simulink model "ADCS_Software"  (R2025b)
settings: Solver=FixedStepDiscrete  StartTime=0.0  StopTime=10.0  RelTol=1e-3
undefined symbols (not defined in the file or in its folder): D1, P
settings Model: OrderFunctionsByDependency=on  Creator=eyrns  LastModifiedBy=eyrns
settings OptimizationCC: DefaultParameterBehavior=Inlined  EnhancedBackFolding=on  PassReuseOutputArgsAs=Individual arguments  ZeroExternalMemoryAtStartup=off  ZeroInternalMemoryAtStartup=off  OptimizeBlockOrder=speed  DifferentSizesBufferReuse=on  OptimizationCustomize=off  EfficientTunableParamExpr=on
settings DebuggingCC: ParameterTunabilityLossMsg=error
settings SFSimCC: MATLABDynamicMemAlloc=off
settings RTWCC: SystemTargetFile=ert.tlc  TemplateMakefile=ert_default_tmf  Description=Embedded Coder
settings CodeAppCC: ForceParamTrailComments=on  IgnoreCustomStorageClasses=off  OperatorAnnotations=on  SimulinkDataObjDesc=on  SFDataObjDesc=on  InsertBlockDesc=on
settings ERTTargetCC: ERTCustomFileTemplate=example_file_process.tlc  TargetLangStandard=C99 (ISO)  GenerateSampleERTMain=on

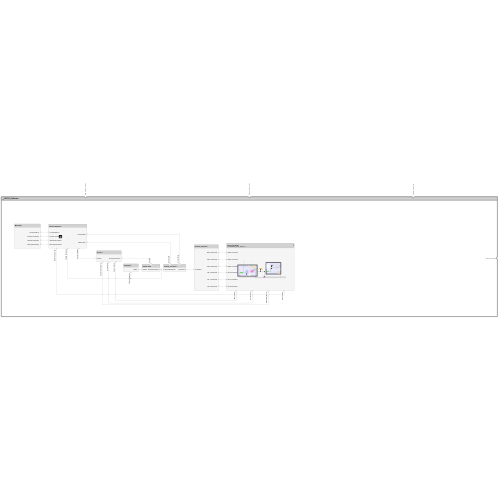
[thumbnail: Simulink's stored preview of the top-level diagram]
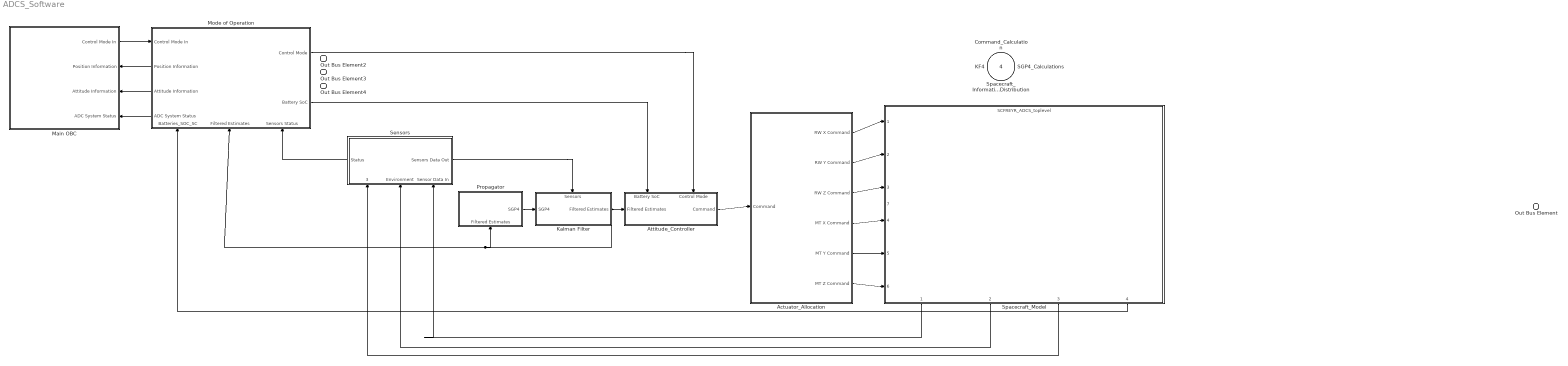
== system ADCS_Software ==
  Spacecraft_Information_Distribution : Inport  OutputFunctionCall=on
  Command_Calculation : Inport  Port=2  OutputFunctionCall=on
  SGP4_Calculations : Inport  Port=3  OutputFunctionCall=on
  KF4 : Inport  Port=4  OutputFunctionCall=on
  Actuator_Allocation : Subsystem
      settings: PortSchema="{\"entries\":[{\"content\":{\"headerSize\":26,\"margin\":15,\"minimumSpacing\":25,\"sides\":[{\"content\":{\"connectorIds\":[\"In1\"]},\"type\":\"ConnectorPlacement.EquallySpacedRectSide\",\"uuid\":\"256b1764-5093-40b4-a299-a96bc66f9c34\"},{\"content\":{\"connectorIds\":[\"Out1\",\"Out2\",\"Out3\",\"Out4\",\"Out5\",\"Out6\"],\"side\":\"RIGHT\"},\"type\":\"ConnectorPlacement.EquallySpacedRectSide\",\"uuid\":\"2deaa205-b527-45f3-83a3-1336b8d1b07d\"},{\"content\":{\"side\":\"TOP\"},\"type\":\"ConnectorPlacement.EquallySpacedRectSide\",\"uuid\":\"e475b6ad-a743-494b-935c-e32dd19b98b9\"}]},\"type\":\"ConnectorPlacement.EquallySpacedConnector\",\"uuid\":\"8ae79be5-f0b0-4f7e-ba91-8d68681c267d\"}],\"packageUris\":[\"http://schema.mathworks.com/mf0/Connector/R2020b\"],\"version\":\"1.0\"}"
  Attitude_Controller : Subsystem
      settings: PortSchema="{\"entries\":[{\"content\":{\"headerSize\":26,\"margin\":15,\"minimumSpacing\":25,\"sides\":[{\"content\":{\"connectorIds\":[\"In2\"]},\"type\":\"ConnectorPlacement.EquallySpacedRectSide\",\"uuid\":\"256b1764-5093-40b4-a299-a96bc66f9c34\"},{\"content\":{\"connectorIds\":[\"Out1\"],\"side\":\"RIGHT\"},\"type\":\"ConnectorPlacement.EquallySpacedRectSide\",\"uuid\":\"2deaa205-b527-45f3-83a3-1336b8d1b07d\"},{\"content\":{\"connectorIds\":[\"In1\",\"In3\"],\"side\":\"TOP\"},\"type\":\"ConnectorPlacement.EquallySpacedRectSide\",\"uuid\":\"e475b6ad-a743-494b-935c-e32dd19b98b9\"},{\"content\":{\"side\":\"BOTTOM\"},\"type\":\"ConnectorPlacement.EquallySpacedRectSide\",\"uuid\":\"40b931e7-0f08-4302-b6a2-74d313a26b2a\"}]},\"type\":\"ConnectorPlacement.EquallySpacedConnector\",\"uuid\":\"8ae79be5-f0b0-4f7e-ba91-8d68681c267d\"}],\"packageUris\":[\"http://schema.mathworks.com/mf0/Connector/R2020b\"],\"version\":\"1.0\"}"
  Kalman Filter : Subsystem
      settings: PortSchema="{\"entries\":[{\"content\":{\"headerSize\":26,\"margin\":15,\"minimumSpacing\":25,\"sides\":[{\"content\":{\"connectorIds\":[\"In1\"]},\"type\":\"ConnectorPlacement.EquallySpacedRectSide\",\"uuid\":\"256b1764-5093-40b4-a299-a96bc66f9c34\"},{\"content\":{\"connectorIds\":[\"Out1\"],\"side\":\"RIGHT\"},\"type\":\"ConnectorPlacement.EquallySpacedRectSide\",\"uuid\":\"2deaa205-b527-45f3-83a3-1336b8d1b07d\"},{\"content\":{\"connectorIds\":[\"In2\"],\"side\":\"TOP\"},\"type\":\"ConnectorPlacement.EquallySpacedRectSide\",\"uuid\":\"e475b6ad-a743-494b-935c-e32dd19b98b9\"}]},\"type\":\"ConnectorPlacement.EquallySpacedConnector\",\"uuid\":\"8ae79be5-f0b0-4f7e-ba91-8d68681c267d\"}],\"packageUris\":[\"http://schema.mathworks.com/mf0/Connector/R2020b\"],\"version\":\"1.0\"}"
  Main OBC : Subsystem
      settings: PortSchema="{\"entries\":[{\"content\":{\"headerSize\":26,\"margin\":15,\"minimumSpacing\":25,\"sides\":[{\"content\":{},\"type\":\"ConnectorPlacement.EquallySpacedRectSide\",\"uuid\":\"3fabc401-0b99-47a6-9b7f-bea42003907c\"},{\"content\":{\"connectorIds\":[\"Out1\",\"In1\",\"In2\",\"In3\"],\"side\":\"RIGHT\"},\"type\":\"ConnectorPlacement.EquallySpacedRectSide\",\"uuid\":\"9a260991-7440-4126-b8d0-233932180f80\"},{\"content\":{\"side\":\"TOP\"},\"type\":\"ConnectorPlacement.EquallySpacedRectSide\",\"uuid\":\"51ce4edb-018b-4faa-870c-da1e497f3f0a\"}]},\"type\":\"ConnectorPlacement.EquallySpacedConnector\",\"uuid\":\"19da0c4b-b9e9-4512-bfc0-b25bda82fb44\"}],\"packageUris\":[\"http://schema.mathworks.com/mf0/Connector/R2020b\"],\"version\":\"1.0\"}"
  Mode of Operation : Subsystem
      settings: PortSchema="{\"entries\":[{\"content\":{\"headerSize\":26,\"margin\":15,\"minimumSpacing\":25,\"sides\":[{\"content\":{\"connectorIds\":[\"In4\",\"Out2\",\"Out3\",\"Out1\"]},\"type\":\"ConnectorPlacement.EquallySpacedRectSide\",\"uuid\":\"256b1764-5093-40b4-a299-a96bc66f9c34\"},{\"content\":{\"connectorIds\":[\"Out4\",\"Out5\"],\"side\":\"RIGHT\"},\"type\":\"ConnectorPlacement.EquallySpacedRectSide\",\"uuid\":\"2deaa205-b527-45f3-83a3-1336b8d1b07d\"},{\"content\":{\"side\":\"TOP\"},\"type\":\"ConnectorPlacement.EquallySpacedRectSide\",\"uuid\":\"e475b6ad-a743-494b-935c-e32dd19b98b9\"},{\"content\":{\"connectorIds\":[\"In3\",\"In1\",\"In2\"],\"side\":\"BOTTOM\"},\"type\":\"ConnectorPlacement.EquallySpacedRectSide\",\"uuid\":\"3bb00a29-bd68-4184-bfee-57dea73dfd28\"}]},\"type\":\"ConnectorPlacement.EquallySpacedConnector\",\"uuid\":\"8ae79be5-f0b0-4f7e-ba91-8d68681c267d\"}],\"packageUris\":[\"http://schema.mathworks.com/mf0/Connector/R2020b\"],\"version\":\"1.0\"}"
  Propagator : Subsystem
      settings: PortSchema="{\"entries\":[{\"content\":{\"headerSize\":26,\"margin\":15,\"minimumSpacing\":25,\"sides\":[{\"content\":{},\"type\":\"ConnectorPlacement.EquallySpacedRectSide\",\"uuid\":\"256b1764-5093-40b4-a299-a96bc66f9c34\"},{\"content\":{\"connectorIds\":[\"Out1\"],\"side\":\"RIGHT\"},\"type\":\"ConnectorPlacement.EquallySpacedRectSide\",\"uuid\":\"2deaa205-b527-45f3-83a3-1336b8d1b07d\"},{\"content\":{\"side\":\"TOP\"},\"type\":\"ConnectorPlacement.EquallySpacedRectSide\",\"uuid\":\"e475b6ad-a743-494b-935c-e32dd19b98b9\"},{\"content\":{\"connectorIds\":[\"In1\"],\"side\":\"BOTTOM\"},\"type\":\"ConnectorPlacement.EquallySpacedRectSide\",\"uuid\":\"f6fae57c-5d41-4f91-83d0-b3c8416bf2e1\"}]},\"type\":\"ConnectorPlacement.EquallySpacedConnector\",\"uuid\":\"8ae79be5-f0b0-4f7e-ba91-8d68681c267d\"}],\"packageUris\":[\"http://schema.mathworks.com/mf0/Connector/R2020b\"],\"version\":\"1.0\"}"
  Sensors : Subsystem
      settings: PortSchema="{\"entries\":[{\"content\":{\"headerSize\":26,\"margin\":15,\"minimumSpacing\":25,\"sides\":[{\"content\":{\"connectorIds\":[\"Out1\"]},\"type\":\"ConnectorPlacement.EquallySpacedRectSide\",\"uuid\":\"256b1764-5093-40b4-a299-a96bc66f9c34\"},{\"content\":{\"connectorIds\":[\"Out2\"],\"side\":\"RIGHT\"},\"type\":\"ConnectorPlacement.EquallySpacedRectSide\",\"uuid\":\"2deaa205-b527-45f3-83a3-1336b8d1b07d\"},{\"content\":{\"side\":\"TOP\"},\"type\":\"ConnectorPlacement.EquallySpacedRectSide\",\"uuid\":\"e475b6ad-a743-494b-935c-e32dd19b98b9\"},{\"content\":{\"connectorIds\":[\"In3\",\"In2\",\"In1\"],\"side\":\"BOTTOM\"},\"type\":\"ConnectorPlacement.EquallySpacedRectSide\",\"uuid\":\"eddd55ac-d30b-499d-8702-4dcff227d580\"}]},\"type\":\"ConnectorPlacement.EquallySpacedConnector\",\"uuid\":\"8ae79be5-f0b0-4f7e-ba91-8d68681c267d\"}],\"packageUris\":[\"http://schema.mathworks.com/mf0/Connector/R2020b\"],\"version\":\"1.0\"}"
  Spacecraft_Model : ModelReference  ModelNameDialog=SCFREYR_ADCS_toplevel.slx  SimulationMode=Normal  ScheduleRates=on  ModelEventPortInfo=P:D1[-2][0][0]  ModelReferenceVersion=9.810
      settings: PortSchema="{\"entries\":[{\"content\":{\"headerSize\":38,\"margin\":15,\"minimumSpacing\":25,\"sides\":[{\"content\":{\"connectorIds\":[\"In1\",\"In2\",\"In3\",\"In4\",\"In5\",\"In6\"]},\"type\":\"ConnectorPlacement.EquallySpacedRectSide\",\"uuid\":\"320dd0f7-d8ad-4694-a861-83cf9b74b79d\"},{\"content\":{\"side\":\"RIGHT\"},\"type\":\"ConnectorPlacement.EquallySpacedRectSide\",\"uuid\":\"325f6c1c-11e2-4f0b-8512-de0a85b49422\"},{\"content\":{\"side\":\"TOP\"},\"type\":\"ConnectorPlacement.EquallySpacedRectSide\",\"uuid\":\"dffe24b9-0a47-4e99-bb19-1bb9da8fb238\"},{\"content\":{\"connectorIds\":[\"Out1\",\"Out2\",\"Out3\",\"Out4\"],\"side\":\"BOTTOM\"},\"type\":\"ConnectorPlacement.EquallySpacedRectSide\",\"uuid\":\"75b260fa-c139-4474-941d-b0acc6263123\"},{\"content\":{\"connectorIds\":[\"In7\"],\"side\":\"HIDDEN\"},\"type\":\"ConnectorPlacement.EquallySpacedRectSide\",\"uuid\":\"2642ed9f-9844-4242-a354-15499d8a4647\"}]},\"type\":\"ConnectorPlacement.EquallySpacedConnector\",\"uuid\":\"23b3e781-752b-4fe3-8111-bbb0bc2569dd\"}],\"packageUris\":[\"http://schema.mathworks.com/mf0/Connector/R2020b\"],\"version\":\"1.0\"}"
  Out Bus Element4 : Outport  PortName=Attitude Information
  Out Bus Element3 : Outport  Port=2  PortName=Position Information
  Out Bus Element2 : Outport  Port=3  PortName=ADC System Status
  Out Bus Element : Outport  Port=4  PortName=Reaction Wheels
  wires:
  Sensors/2(Sensors Data Out) -> Kalman Filter/2(Sensors)
  Propagator/1(SGP4) -> Kalman Filter/1(SGP4)
  Kalman Filter/1(Filtered Estimates) -> Mode of Operation/1(Filtered Estimates), Propagator/1(Filtered Estimates), Attitude_Controller/2(Filtered Estimates)
  Attitude_Controller/1(Command) -> Actuator_Allocation/1(Command)
  Mode of Operation/4(Control Mode) -> Attitude_Controller/3(Control Mode)
  Mode of Operation/5(Battery SoC) -> Attitude_Controller/1(Battery SoC)
  Mode of Operation/1(ADC System Status) -> Main OBC/3(ADC System Status)
  Mode of Operation/2(Position Information) -> Main OBC/1(Position Information)
  Mode of Operation/3(Attitude Information) -> Main OBC/2(Attitude Information)
  Sensors/1(Status) -> Mode of Operation/2(Sensors Status)
  Actuator_Allocation/1(RW X Command) -> Spacecraft_Model/1
  Actuator_Allocation/2(RW Y Command) -> Spacecraft_Model/2
  Actuator_Allocation/3(RW Z Command) -> Spacecraft_Model/3
  Actuator_Allocation/4(MT X Command) -> Spacecraft_Model/4
  Actuator_Allocation/5(MT Y Command) -> Spacecraft_Model/5
  Actuator_Allocation/6(MT Z Command) -> Spacecraft_Model/6
  Spacecraft_Model/1 -> Sensors/1(Sensor Data In)
  Spacecraft_Model/2 -> Sensors/2(Environment)
  Spacecraft_Model/3 -> Sensors/3(Spacecraft Dynamics)
  Spacecraft_Model/4 -> Mode of Operation/3(Batteries_SOC_SC)
  Main OBC/1(Control Mode In) -> Mode of Operation/4(Control Mode In)

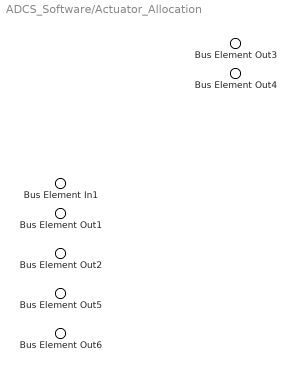
== system ADCS_Software/Actuator_Allocation ==
  Bus Element In1 : Inport  PortName=Command
  Bus Element Out1 : Outport  PortName=RW X Command
  Bus Element Out3 : Outport  Port=2  PortName=RW Y Command
  Bus Element Out4 : Outport  Port=3  PortName=RW Z Command
  Bus Element Out2 : Outport  Port=4  PortName=MT X Command
  Bus Element Out5 : Outport  Port=5  PortName=MT Y Command
  Bus Element Out6 : Outport  Port=6  PortName=MT Z Command

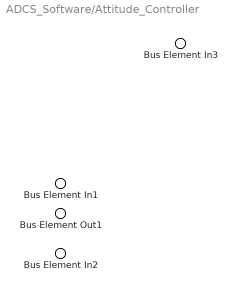
== system ADCS_Software/Attitude_Controller ==
  Bus Element In3 : Inport  PortName=Battery SoC
  Bus Element In1 : Inport  Port=2  PortName=Filtered Estimates
  Bus Element In2 : Inport  Port=3  PortName=Control Mode
  Bus Element Out1 : Outport  PortName=Command

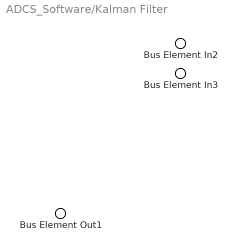
== system ADCS_Software/Kalman Filter ==
  Bus Element In3 : Inport  PortName=SGP4
  Bus Element In2 : Inport  Port=2  PortName=Sensors
  Bus Element Out1 : Outport  PortName=Filtered Estimates

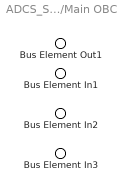
== system ADCS_Software/Main OBC ==
  Bus Element In1 : Inport  PortName=Position Information
  Bus Element In2 : Inport  Port=2  PortName=Attitude Information
  Bus Element In3 : Inport  Port=3  PortName=ADC System Status
  Bus Element Out1 : Outport  PortName=Control Mode In

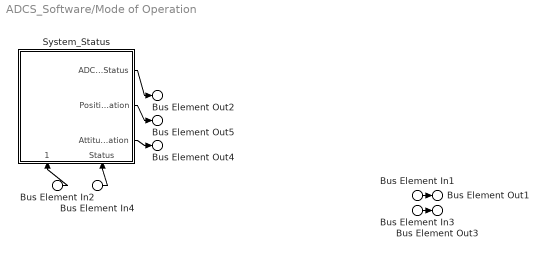
== system ADCS_Software/Mode of Operation ==
  Bus Element In2 : Inport  PortName=Filtered Estimates
  Bus Element In4 : Inport  Port=2  PortName=Sensors Status
  Bus Element In3 : Inport  Port=3  PortName=Batteries_SOC_SC
  Bus Element In1 : Inport  Port=4  PortName=Control Mode In
  System_Status : Subsystem
      settings: PortSchema="{\"entries\":[{\"content\":{\"headerSize\":26,\"margin\":15,\"minimumSpacing\":25,\"sides\":[{\"content\":{},\"type\":\"ConnectorPlacement.EquallySpacedRectSide\",\"uuid\":\"256b1764-5093-40b4-a299-a96bc66f9c34\"},{\"content\":{\"connectorIds\":[\"Out1\",\"Out2\",\"Out3\"],\"side\":\"RIGHT\"},\"type\":\"ConnectorPlacement.EquallySpacedRectSide\",\"uuid\":\"2deaa205-b527-45f3-83a3-1336b8d1b07d\"},{\"content\":{\"side\":\"TOP\"},\"type\":\"ConnectorPlacement.EquallySpacedRectSide\",\"uuid\":\"e475b6ad-a743-494b-935c-e32dd19b98b9\"},{\"content\":{\"connectorIds\":[\"In1\",\"In2\"],\"side\":\"BOTTOM\"},\"type\":\"ConnectorPlacement.EquallySpacedRectSide\",\"uuid\":\"3e6c55d2-1ccb-451b-ace1-31b90a933923\"}]},\"type\":\"ConnectorPlacement.EquallySpacedConnector\",\"uuid\":\"8ae79be5-f0b0-4f7e-ba91-8d68681c267d\"}],\"packageUris\":[\"http://schema.mathworks.com/mf0/Connector/R2020b\"],\"version\":\"1.0\"}"
  Bus Element Out2 : Outport  PortName=ADC System Status
  Bus Element Out5 : Outport  Port=2  PortName=Position Information
  Bus Element Out4 : Outport  Port=3  PortName=Attitude Information
  Bus Element Out1 : Outport  Port=4  PortName=Control Mode
  Bus Element Out3 : Outport  Port=5  PortName=Battery SoC
  wires:
  Bus Element In1/1 -> Bus Element Out1/1
  Bus Element In3/1 -> Bus Element Out3/1
  Bus Element In2/1 -> System_Status/1(Filtered Estimates)
  System_Status/1(ADC System Status) -> Bus Element Out2/1
  System_Status/2(Position Information) -> Bus Element Out5/1
  System_Status/3(Attitude Information) -> Bus Element Out4/1
  Bus Element In4/1 -> System_Status/2(Status)

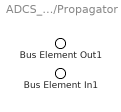
== system ADCS_Software/Propagator ==
  Bus Element In1 : Inport  PortName=Filtered Estimates
  Bus Element Out1 : Outport  PortName=SGP4

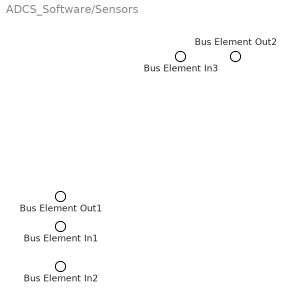
== system ADCS_Software/Sensors ==
  Bus Element In3 : Inport  PortName=Sensor Data In
  Bus Element In1 : Inport  Port=2  PortName=Environment
  Bus Element In2 : Inport  Port=3  PortName=Spacecraft Dynamics
  Bus Element Out2 : Outport  PortName=Status
  Bus Element Out1 : Outport  Port=2  PortName=Sensors Data Out

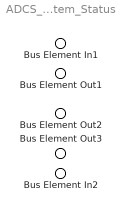
== system ADCS_Software/Mode of Operation/System_Status ==
  Bus Element In1 : Inport  PortName=Filtered Estimates
  Bus Element In2 : Inport  Port=2  PortName=Status
  Bus Element Out1 : Outport  PortName=ADC System Status
  Bus Element Out2 : Outport  Port=2  PortName=Position Information
  Bus Element Out3 : Outport  Port=3  PortName=Attitude Information
